simulink model "ZweiPunktRegler"  (R2019b)
settings: Solver=VariableStepAuto  StartTime=0.0  StopTime=20  RelTol=1e-3
settings Model: Creator=Ossmann  LastModifiedBy=Ossmann
settings SFSimCC: CustomCodeUndefinedFunction=UseInterfaceOnly

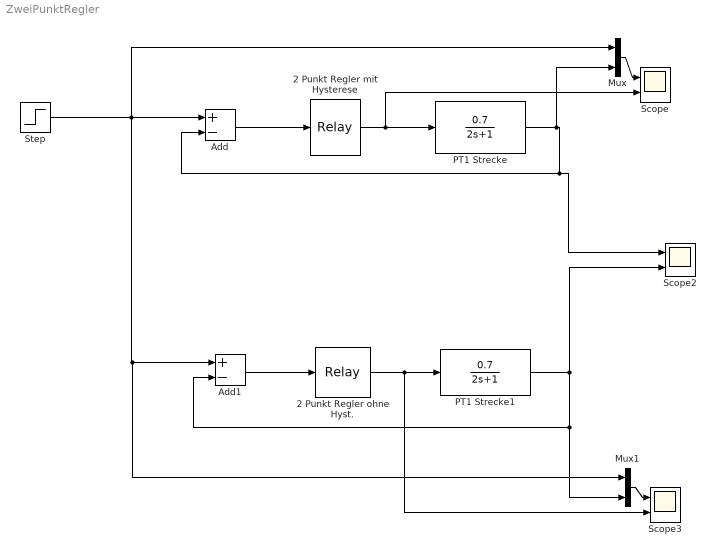
== system ZweiPunktRegler ==
  2 Punkt Regler mit Hysterese : Relay  OnSwitchValue=0.2  OffSwitchValue=-0.2  OnOutputValue=3
  2 Punkt Regler ohne Hyst. : Relay  OnSwitchValue=0.001  OffSwitchValue=-0.001  OnOutputValue=3
  Add : Sum  Inputs=+-
  Add1 : Sum  Inputs=+-
  Mux : Mux  Inputs=2
  Mux1 : Mux  Inputs=2
  PT1 Strecke : TransferFcn  Numerator=0.7  Denominator=[2 1]
  PT1 Strecke1 : TransferFcn  Numerator=0.7  Denominator=[2 1]
  Scope : Scope  NumInputPorts=2
  Scope2 : Scope  NumInputPorts=2
  Scope3 : Scope  NumInputPorts=2
  Step : Step  After=1.5  SampleTime=0
  wires:
  PT1 Strecke/1 -> Mux/2, Add/2, Scope2/1
  Add/1 -> 2 Punkt Regler mit Hysterese/1
  2 Punkt Regler mit Hysterese/1 -> Scope/2, PT1 Strecke/1
  Add1/1 -> 2 Punkt Regler ohne Hyst./1
  PT1 Strecke1/1 -> Scope2/2, Mux1/2, Add1/2
  Step/1 -> Mux/1, Add/1, Mux1/1, Add1/1
  Mux/1 -> Scope/1
  Mux1/1 -> Scope3/1
  2 Punkt Regler ohne Hyst./1 -> Scope3/2, PT1 Strecke1/1
